simulink model "project_589"  (R2020b)
settings: Solver=VariableStepAuto  StartTime=0.0  StopTime=2  RelTol=1e-3
libraries: powerlib x25, powerlib_meascontrol x8, simulink x7, re_lib x2, fillib x1
(part 2 of 2)

== matlab function project_589/MATLAB Function6 ==
  settings: updateMethod=DISCRETE
  data: Vpv input; choice output; xhat input; y output; Ipv input; Ipv_plus_on input; Ipv_plus_off input; debug1 output; debug2 output
function [choice, y, debug1, debug2]= fcn(Vpv, xhat, Ipv, Ipv_plus_on, Ipv_plus_off)
% Vout=xhat(4);

%This module contains the MPC-MPPT Control Algorithm

%The MPC module follows the flow chart of Fig. 8 in Referenced Research Paper

%This MATLAB fn block's settings have been changed to have a sampling rate
%of 15uS instead of being continous sample mode


%prevent crazy simulation transients from breaking the algorithm:
if (Ipv > 10)
    Ipv = 1;
end

persistent DC;
if isempty(DC)
    DC = 0;
end

persistent Vpv_t_1; %previous Vpv Sample
if isempty(Vpv_t_1)
    Vpv_t_1 = 0;
end
persistent Ipv_t_1; %previous Ipv Sample
if isempty(Ipv_t_1)
    Ipv_t_1 = 0;
end
persistent Dpv_t_1; % Iref (output) value from what is now 2 timesteps ago
if isempty(Dpv_t_1)
    Dpv_t_1 = 0;
end
persistent Dpv;  %Previous / Most recent Iref (output) Calc
if isempty(Dpv)
    Dpv = 0;
end

Ts = 15e-6; %sample rate
L = 3e-3; %inductance


delta_V = Vpv - Vpv_t_1;
delta_I = Ipv - Ipv_t_1;
delta_D = Dpv - Dpv_t_1;


%fixed vs adaptive
scale_factor_C = 10; %increase for larger output increments/swings
 Z =.001; %fixed 
%Z = scale_factor_C * abs(delta_I * delta_D); %adaptive

% custom adaptive to fix issues with no change causing 0 step size
 adapZ = scale_factor_C * abs(delta_I * delta_D);
% if(adapZ > .1)
%     Z = .1;
% elseif(adapZ > .001)
%     Z = adapZ;
% else
%     Z = .001;
% end

Ipred_1 = Ipv_plus_on;
Ipred_0 = Ipv_plus_off;
%Ipred_1 = Ipv + 2*(Ts/L) * Vpv; %MPC prediction for switch = 1
%Ipred_0 = Ipv + (Ts/(2*L)* (Vpv - Vout)); %MPC prediction for switch = 0 

if delta_V == 0 %Inc. Cond. Algo to determine Iref
    if delta_I == 0 
        Iref = Dpv; choice = 0;
    else
        if delta_I > 0
            Iref = Dpv - Z; choice = 1;
        else
            Iref = Dpv + Z; choice = 2;
        end
    end
else
    if (Ipv + (delta_I/delta_V) * Vpv) == 0
        Iref = Dpv; choice = 3;
    else
        if (Ipv + (delta_I/delta_V) * Vpv) > 0
            Iref = Dpv - Z; choice = 4;
        else
            Iref = Dpv + Z; choice = 5;
        end
    end
end

G1 = abs(Iref - Ipred_1); %Optimize MPC by applying Iref
G0 = abs(Iref - Ipred_0);
if G1 < G0
    DC = DC + .0005;
else
    DC = DC - .0005;
end

if (DC < 0)
    DC = 0;
end
if (DC > 1)
    DC = 1;
end

if (Iref < 0)
    Iref = .001;
end
%test = Ipv + (delta_I/delta_V) * Vpv;
test =  delta_V;
%update static variables here:
Vpv_t_1 = Vpv; %previous Vpv Sample
Ipv_t_1 = Ipv; %previous Ipv Sample
Dpv_t_1 = Dpv; % Iref (output) value from what is now 2 timesteps ago
Dpv = Iref;  %Previous / Most recent Iref (output) Calc

y = DC;

%debug purposes:
debug1 = Iref;
debug2 = delta_I/delta_V;

== matlab function project_589/MATLAB Function7 ==
  settings: updateMethod=DISCRETE
  data: Y output; u input; num_ones output
function [Y, num_ones] = fcn(u)

persistent A;
if isempty(A)
    A = zeros(1,10);
end

A = circshift(A,1);
A(1,1) = u;

num_ones = 0;
% num_zeros = 0;
for i=1:1:10
    if(A(1,i)== 1)
        num_ones = num_ones + 1;
    end
end
% for i=1:1:20
%     if(A(i)== 0)
%         num_zeros = num_zeros + 1;
%     end
% end

Tsample = 15e-6;
Ts = 10*Tsample;
D = num_ones*Tsample / Ts;
Y = D;

== matlab function project_589/MATLAB Function8 ==
  settings: updateMethod=DISCRETE
  data: Y output; Vpv input; Ipv input
function Y= fcn(Vpv, Ipv)

persistent DC;
if isempty(DC)
    DC = 0;
end

persistent Vpv_t_1;
if isempty(Vpv_t_1)
    Vpv_t_1 = 0;
end
persistent Ipv_t_1;
if isempty(Ipv_t_1)
    Ipv_t_1 = 0;
end

Delta_V = Vpv - Vpv_t_1;
Delta_I = Ipv - Ipv_t_1;

if (Delta_V == 0 && Delta_I == 0) DC = DC; 
elseif (Delta_V == 0 && Delta_I > 0) DC = DC - .0005; 
elseif (Delta_V == 0 && Delta_I < 0) DC = DC + .0005; 
elseif (Delta_V ~= 0 && Delta_I/Delta_V == -Ipv/Vpv) DC = DC; 
elseif (Delta_V ~= 0 && Delta_I/Delta_V ~= -Ipv/Vpv && Delta_I/Delta_V > -Ipv/Vpv) DC = DC - .0005; 
elseif (Delta_V ~= 0 && Delta_I/Delta_V ~= -Ipv/Vpv && Delta_I/Delta_V < -Ipv/Vpv) DC = DC + .0005; 
end
% Z = .001;
% if Delta_V == 0 %Inc. Cond. Algo to determin DC
%     if delta_I == 0 
%         DC = DC; choice = 0;
%     else
%         if delta_I > 0
%             DC = DC - Z; choice = 1;
%         else
%             DC = DC + Z; choice = 2;
%         end
%     end
% else
%     if (Ipv + (delta_I/Delta_V) * Vpv) == 0
%         DC = DC; choice = 3;
%     else
%         if (Ipv + (delta_I/Delta_V) * Vpv) > 0
%             DC = DC - Z; choice = 4;
%         else
%             DC = DC + Z; choice = 5;
%         end
%     end
% end


if(DC < 0) DC = 0; end
if(DC > 1) DC = 1; end

Vpv_t_1 = Vpv;
Ipv_t_1 = Ipv;
Y = DC;
